simulink model "PTC_MBDS_StringDelete_Sample"  (R2013a)
settings: Solver=FixedStepDiscrete  StartTime=0.0  StopTime=100  FixedStep=0.02  RelTol=1e-3
libraries: PTC_MBDS_LIB x12, simulink_extras x1
settings Model: Creator=uidl7367  LastModifiedBy=sundeep.tuteja
settings DataIOCC: SignalLoggingSaveFormat=ModelDataLogs
settings OptimizationCC: ExpressionDepthLimit=2147483647  InitFltsAndDblsToZero=on
settings DebuggingCC: SaveWithParameterizedLinksMsg=none  SignalResolutionControl=TryResolveAllWithWarning  InheritedTsInSrcMsg=none  MultiTaskDSMMsg=warning  MultiTaskCondExecSysMsg=none  FcnCallInpInsideContextMsg=UseLocalSettings  StrictBusMsg=Warning
settings RTWCC: IncludeERTFirstTime=on
settings GRTTargetCC: TargetFcnLib=ansi_tfl_tmw.mat  CombineOutputUpdateFcns=off  GRTInterface=on

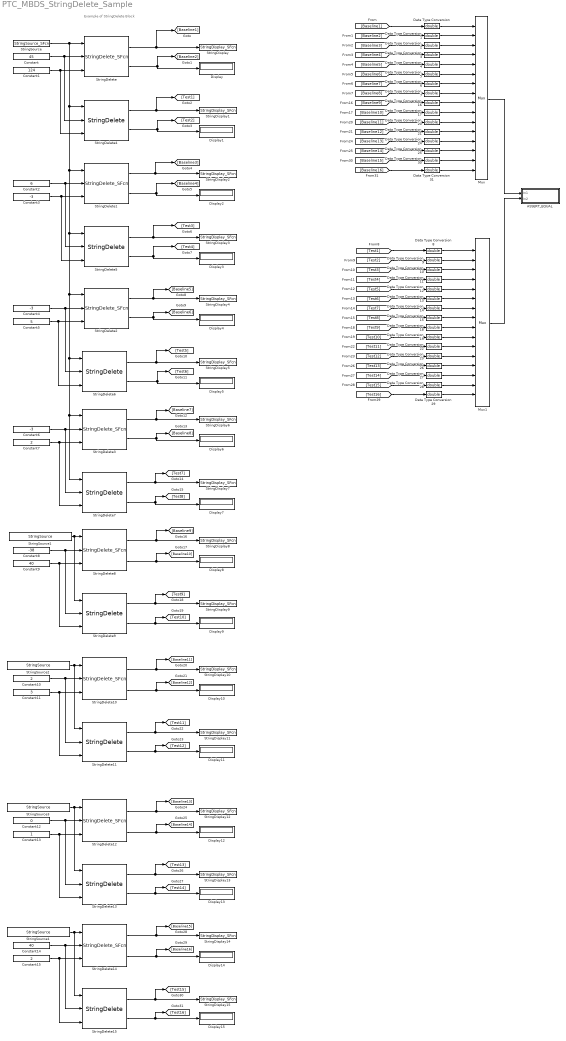
== system PTC_MBDS_StringDelete_Sample ==
  note: Example of StringDelete Block
  ASSERT_EQUAL : Subsystem
  Constant : Constant  InitFcn=|  Value=45  VectorParams1D=off  OutDataTypeStr=int8
      | if(exist('MBDS_BlockCallback', 'file'))
      |    MBDS_BlockCallback('Update', gcb);  
      | end
  Constant1 : Constant  InitFcn=|  Value=124  VectorParams1D=off  OutDataTypeStr=int8
      | if(exist('MBDS_BlockCallback', 'file'))
      |    MBDS_BlockCallback('Update', gcb);  
      | end
  Constant10 : Constant  InitFcn=|  Value=2  VectorParams1D=off  OutDataTypeStr=int8
      | if(exist('MBDS_BlockCallback', 'file'))
      |    MBDS_BlockCallback('Update', gcb);  
      | end
  Constant11 : Constant  InitFcn=|  Value=3  VectorParams1D=off  OutDataTypeStr=int8
      | if(exist('MBDS_BlockCallback', 'file'))
      |    MBDS_BlockCallback('Update', gcb);  
      | end
  Constant12 : Constant  InitFcn=|  Value=0  VectorParams1D=off  OutDataTypeStr=int8
      | if(exist('MBDS_BlockCallback', 'file'))
      |    MBDS_BlockCallback('Update', gcb);  
      | end
  Constant13 : Constant  InitFcn=|  VectorParams1D=off  OutDataTypeStr=int8
      | if(exist('MBDS_BlockCallback', 'file'))
      |    MBDS_BlockCallback('Update', gcb);  
      | end
  Constant14 : Constant  InitFcn=|  Value=40  VectorParams1D=off  OutDataTypeStr=int8
      | if(exist('MBDS_BlockCallback', 'file'))
      |    MBDS_BlockCallback('Update', gcb);  
      | end
  Constant15 : Constant  InitFcn=|  Value=2  VectorParams1D=off  OutDataTypeStr=int8
      | if(exist('MBDS_BlockCallback', 'file'))
      |    MBDS_BlockCallback('Update', gcb);  
      | end
  Constant2 : Constant  InitFcn=|  Value=6  VectorParams1D=off  OutDataTypeStr=int8
      | if(exist('MBDS_BlockCallback', 'file'))
      |    MBDS_BlockCallback('Update', gcb);  
      | end
  Constant3 : Constant  InitFcn=|  Value=-3  VectorParams1D=off  OutDataTypeStr=int8
      | if(exist('MBDS_BlockCallback', 'file'))
      |    MBDS_BlockCallback('Update', gcb);  
      | end
  Constant4 : Constant  InitFcn=|  Value=-3  VectorParams1D=off  OutDataTypeStr=int8
      | if(exist('MBDS_BlockCallback', 'file'))
      |    MBDS_BlockCallback('Update', gcb);  
      | end
  Constant5 : Constant  InitFcn=|  Value=5  VectorParams1D=off  OutDataTypeStr=int8
      | if(exist('MBDS_BlockCallback', 'file'))
      |    MBDS_BlockCallback('Update', gcb);  
      | end
  Constant6 : Constant  InitFcn=|  Value=-3  VectorParams1D=off  OutDataTypeStr=int8
      | if(exist('MBDS_BlockCallback', 'file'))
      |    MBDS_BlockCallback('Update', gcb);  
      | end
  Constant7 : Constant  InitFcn=|  Value=2  VectorParams1D=off  OutDataTypeStr=int8
      | if(exist('MBDS_BlockCallback', 'file'))
      |    MBDS_BlockCallback('Update', gcb);  
      | end
  Constant8 : Constant  InitFcn=|  Value=-38  VectorParams1D=off  OutDataTypeStr=int8
      | if(exist('MBDS_BlockCallback', 'file'))
      |    MBDS_BlockCallback('Update', gcb);  
      | end
  Constant9 : Constant  InitFcn=|  Value=40  VectorParams1D=off  OutDataTypeStr=int8
      | if(exist('MBDS_BlockCallback', 'file'))
      |    MBDS_BlockCallback('Update', gcb);  
      | end
  Data Type Conversion{,1..31} (32 alike) : DataTypeConversion  OutDataTypeStr=double
  Display{,1..15} (16 alike) : Display
  Mux : Mux  Inputs=16
  Mux1 : Mux  Inputs=16
  StringDelete : S-Function  InitFcn=|  FunctionName=StringDelete_SFcn  Parameters=boolean(ENO_Enabled), uint16(MaxStringLength)  EnableBusSupport=off  mask(StringDelete){MBDS_LibraryBlock=on, ENO_Enabled=on, MBDS_BlockVersion=05.40}
      | if(exist('MBDS_BlockCallback', 'file'))
      |    MBDS_BlockCallback('Update', gcb);
      | end
      mask prompts: MBDS_LibraryBlock "MBDS Library Block"; ENO_Enabled "Show ENO port"; MBDS_BlockVersion "Block version:"
      mask help: Removes a part of the string at input port In. The first character to be removed is given by P, the number of characters to be removed is given by L.
      mask init:
      | MBDS_BlockCallback('Copy', gcb);
      | MaxStringLength = 1 + GetStringLen();
      | maskdisplay = ['disp(''Delete'')' 10];
      | maskdisplay = [maskdisplay 'port_label(''input'', 1, ''In'')' 10];
      | maskdisplay = [maskdisplay 'port_label(''input'', 2, ''L'')' 10];
      | maskdisplay = [maskdisplay 'port_label(''input'', 3, ''P'')' 10];
      | maskdisplay = [maskdisplay 'port_label(''output'', 1, ''Out'')' 10];
      | if(ENO_Enabled)
      | 	maskdisplay = [maskdisplay 'port_label(''output'', 2, ''ENO'')' 10];
      | end
      | set_param(gcbh, 'maskdisplay', maskdisplay)
      mask Help: eval(['open([workdir(''Library_Dir:''),''\Blockset\Help\'',get_param(gcb,''MaskType''),''.html''])'])
      mask Display:
      | disp('Delete')
      | port_label('input', 1, 'In')
      | port_label('input', 2, 'L')
      | port_label('input', 3, 'P')
      | port_label('output', 1, 'Out')
      | port_label('output', 2, 'ENO')
  StringDelete1 : S-Function  InitFcn=|  FunctionName=StringDelete_SFcn  Parameters=boolean(ENO_Enabled), uint16(MaxStringLength)  EnableBusSupport=off  mask(StringDelete){MBDS_LibraryBlock=on, ENO_Enabled=on, MBDS_BlockVersion=05.40}
      | if(exist('MBDS_BlockCallback', 'file'))
      |    MBDS_BlockCallback('Update', gcb);
      | end
      mask prompts: MBDS_LibraryBlock "MBDS Library Block"; ENO_Enabled "Show ENO port"; MBDS_BlockVersion "Block version:"
      mask help: Removes a part of the string at input port In. The first character to be removed is given by P, the number of characters to be removed is given by L.
      mask init: same as PTC_MBDS_StringDelete_Sample/StringDelete
      mask Help: eval(['open([workdir(''Library_Dir:''),''\Blockset\Help\'',get_param(gcb,''MaskType''),''.html''])'])
      mask Display:
      | disp('Delete')
      | port_label('input', 1, 'In')
      | port_label('input', 2, 'L')
      | port_label('input', 3, 'P')
      | port_label('output', 1, 'Out')
      | port_label('output', 2, 'ENO')
  StringDelete10 : S-Function  InitFcn=|  FunctionName=StringDelete_SFcn  Parameters=boolean(ENO_Enabled), uint16(MaxStringLength)  EnableBusSupport=off  mask(StringDelete){MBDS_LibraryBlock=on, ENO_Enabled=on, MBDS_BlockVersion=05.32}
      | if(exist('MBDS_BlockCallback', 'file'))
      |    MBDS_BlockCallback('Update', gcb);
      | end
      mask prompts: MBDS_LibraryBlock "MBDS Library Block"; ENO_Enabled "Show ENO port"; MBDS_BlockVersion "Block version:"
      mask help: Removes a part of the string at input port In. The first character to be removed is given by P, the number of characters to be removed is given by L.
      mask init: same as PTC_MBDS_StringDelete_Sample/StringDelete
      mask Help: eval(['open([workdir(''Library_Dir:''),''\Blockset\Help\'',get_param(gcb,''MaskType''),''.html''])'])
      mask Display:
      | disp('Delete')
      | port_label('input', 1, 'In')
      | port_label('input', 2, 'L')
      | port_label('input', 3, 'P')
      | port_label('output', 1, 'Out')
      | port_label('output', 2, 'ENO')
  StringDelete{4..7,9,11,13,15} (8 alike) : PTC_MBDS_LIB/MBDS Standard Library/Extended Operations/String Operations/StringDelete  ENO_Enabled=on  MaxStringLength=PTC_MBDS_MaxStringLength_Fcn  PTC_MBDS_BlockVersion=5.32  PTC_BlockType=PTC_MBDS_StringDelete
  StringDelete12 : S-Function  InitFcn=|  FunctionName=StringDelete_SFcn  Parameters=boolean(ENO_Enabled), uint16(MaxStringLength)  EnableBusSupport=off  mask(StringDelete){MBDS_LibraryBlock=on, ENO_Enabled=on, MBDS_BlockVersion=05.32}
      | if(exist('MBDS_BlockCallback', 'file'))
      |    MBDS_BlockCallback('Update', gcb);
      | end
      mask prompts: MBDS_LibraryBlock "MBDS Library Block"; ENO_Enabled "Show ENO port"; MBDS_BlockVersion "Block version:"
      mask help: Removes a part of the string at input port In. The first character to be removed is given by P, the number of characters to be removed is given by L.
      mask init: same as PTC_MBDS_StringDelete_Sample/StringDelete
      mask Help: eval(['open([workdir(''Library_Dir:''),''\Blockset\Help\'',get_param(gcb,''MaskType''),''.html''])'])
      mask Display:
      | disp('Delete')
      | port_label('input', 1, 'In')
      | port_label('input', 2, 'L')
      | port_label('input', 3, 'P')
      | port_label('output', 1, 'Out')
      | port_label('output', 2, 'ENO')
  StringDelete14 : S-Function  InitFcn=|  FunctionName=StringDelete_SFcn  Parameters=boolean(ENO_Enabled), uint16(MaxStringLength)  EnableBusSupport=off  mask(StringDelete){MBDS_LibraryBlock=on, ENO_Enabled=on, MBDS_BlockVersion=05.32}
      | if(exist('MBDS_BlockCallback', 'file'))
      |    MBDS_BlockCallback('Update', gcb);
      | end
      mask prompts: MBDS_LibraryBlock "MBDS Library Block"; ENO_Enabled "Show ENO port"; MBDS_BlockVersion "Block version:"
      mask help: Removes a part of the string at input port In. The first character to be removed is given by P, the number of characters to be removed is given by L.
      mask init: same as PTC_MBDS_StringDelete_Sample/StringDelete
      mask Help: eval(['open([workdir(''Library_Dir:''),''\Blockset\Help\'',get_param(gcb,''MaskType''),''.html''])'])
      mask Display:
      | disp('Delete')
      | port_label('input', 1, 'In')
      | port_label('input', 2, 'L')
      | port_label('input', 3, 'P')
      | port_label('output', 1, 'Out')
      | port_label('output', 2, 'ENO')
  StringDelete2 : S-Function  InitFcn=|  FunctionName=StringDelete_SFcn  Parameters=boolean(ENO_Enabled), uint16(MaxStringLength)  EnableBusSupport=off  mask(StringDelete){MBDS_LibraryBlock=on, ENO_Enabled=on, MBDS_BlockVersion=05.40}
      | if(exist('MBDS_BlockCallback', 'file'))
      |    MBDS_BlockCallback('Update', gcb);
      | end
      mask prompts: MBDS_LibraryBlock "MBDS Library Block"; ENO_Enabled "Show ENO port"; MBDS_BlockVersion "Block version:"
      mask help: Removes a part of the string at input port In. The first character to be removed is given by P, the number of characters to be removed is given by L.
      mask init: same as PTC_MBDS_StringDelete_Sample/StringDelete
      mask Help: eval(['open([workdir(''Library_Dir:''),''\Blockset\Help\'',get_param(gcb,''MaskType''),''.html''])'])
      mask Display:
      | disp('Delete')
      | port_label('input', 1, 'In')
      | port_label('input', 2, 'L')
      | port_label('input', 3, 'P')
      | port_label('output', 1, 'Out')
      | port_label('output', 2, 'ENO')
  StringDelete3 : S-Function  InitFcn=|  FunctionName=StringDelete_SFcn  Parameters=boolean(ENO_Enabled), uint16(MaxStringLength)  EnableBusSupport=off  mask(StringDelete){MBDS_LibraryBlock=on, ENO_Enabled=on, MBDS_BlockVersion=05.40}
      | if(exist('MBDS_BlockCallback', 'file'))
      |    MBDS_BlockCallback('Update', gcb);
      | end
      mask prompts: MBDS_LibraryBlock "MBDS Library Block"; ENO_Enabled "Show ENO port"; MBDS_BlockVersion "Block version:"
      mask help: Removes a part of the string at input port In. The first character to be removed is given by P, the number of characters to be removed is given by L.
      mask init: same as PTC_MBDS_StringDelete_Sample/StringDelete
      mask Help: eval(['open([workdir(''Library_Dir:''),''\Blockset\Help\'',get_param(gcb,''MaskType''),''.html''])'])
      mask Display:
      | disp('Delete')
      | port_label('input', 1, 'In')
      | port_label('input', 2, 'L')
      | port_label('input', 3, 'P')
      | port_label('output', 1, 'Out')
      | port_label('output', 2, 'ENO')
  StringDelete8 : S-Function  InitFcn=|  FunctionName=StringDelete_SFcn  Parameters=boolean(ENO_Enabled), uint16(MaxStringLength)  EnableBusSupport=off  mask(StringDelete){MBDS_LibraryBlock=on, ENO_Enabled=on, MBDS_BlockVersion=05.32}
      | if(exist('MBDS_BlockCallback', 'file'))
      |    MBDS_BlockCallback('Update', gcb);
      | end
      mask prompts: MBDS_LibraryBlock "MBDS Library Block"; ENO_Enabled "Show ENO port"; MBDS_BlockVersion "Block version:"
      mask help: Removes a part of the string at input port In. The first character to be removed is given by P, the number of characters to be removed is given by L.
      mask init: same as PTC_MBDS_StringDelete_Sample/StringDelete
      mask Help: eval(['open([workdir(''Library_Dir:''),''\Blockset\Help\'',get_param(gcb,''MaskType''),''.html''])'])
      mask Display:
      | disp('Delete')
      | port_label('input', 1, 'In')
      | port_label('input', 2, 'L')
      | port_label('input', 3, 'P')
      | port_label('output', 1, 'Out')
      | port_label('output', 2, 'ENO')
  StringDisplay : M-S-Function  InitFcn=|  FunctionName=StringDisplay_SFcn  Parameters=MaxRowCount  mask(StringDisplay){MBDS_LibraryBlock=on, MaxRowCount=1, MBDS_BlockVersion=05.20}
      | if(exist('MBDS_BlockCallback', 'file'))
      |    MBDS_BlockCallback('Update', gcb);
      | end
      mask prompts: MBDS_LibraryBlock "MBDS Library Block"; MaxRowCount "Maximum number of rows displayed (min. 1):"; MBDS_BlockVersion "Block version:"
      mask help: The string display block shows an uint8 array as ASCII strings on the block mask.
      mask init:
      | MBDS_BlockCallback('Copy', gcb);
      mask Help: eval(['open([workdir(''Library_Dir:''),''\Blockset\Help\'',get_param(gcb,''MaskType''),''.html''])'])
      mask Callback MaxRowCount:
      | if(str2double(get_param(gcb, 'MaxRowCount')) < 1)
      |    set_param(gcb, 'MaxRowCount', '1');
      | end
      mask Display: text(0.05,0.5,'40_character_string_00000000000000000000','horizontalAlignment','left','verticalAlignment','middle')
  StringDisplay1 : M-S-Function  InitFcn=|  FunctionName=StringDisplay_SFcn  Parameters=MaxRowCount  mask(StringDisplay){MBDS_LibraryBlock=on, MaxRowCount=1, MBDS_BlockVersion=05.20}
      | if(exist('MBDS_BlockCallback', 'file'))
      |    MBDS_BlockCallback('Update', gcb);
      | end
      mask prompts: MBDS_LibraryBlock "MBDS Library Block"; MaxRowCount "Maximum number of rows displayed (min. 1):"; MBDS_BlockVersion "Block version:"
      mask help: The string display block shows an uint8 array as ASCII strings on the block mask.
      mask init:
      | MBDS_BlockCallback('Copy', gcb);
      mask Help: eval(['open([workdir(''Library_Dir:''),''\Blockset\Help\'',get_param(gcb,''MaskType''),''.html''])'])
      mask Callback MaxRowCount:
      | if(str2double(get_param(gcb, 'MaxRowCount')) < 1)
      |    set_param(gcb, 'MaxRowCount', '1');
      | end
      mask Display: text(0.05,0.5,'40_character_string_00000000000000000000','horizontalAlignment','left','verticalAlignment','middle')
  StringDisplay10 : M-S-Function  InitFcn=|  FunctionName=StringDisplay_SFcn  Parameters=MaxRowCount  mask(StringDisplay){MBDS_LibraryBlock=on, MaxRowCount=1, MBDS_BlockVersion=05.20}
      | if(exist('MBDS_BlockCallback', 'file'))
      |    MBDS_BlockCallback('Update', gcb);
      | end
      mask prompts: MBDS_LibraryBlock "MBDS Library Block"; MaxRowCount "Maximum number of rows displayed (min. 1):"; MBDS_BlockVersion "Block version:"
      mask help: The string display block shows an uint8 array as ASCII strings on the block mask.
      mask init:
      | MBDS_BlockCallback('Copy', gcb);
      mask Help: eval(['open([workdir(''Library_Dir:''),''\Blockset\Help\'',get_param(gcb,''MaskType''),''.html''])'])
      mask Callback MaxRowCount:
      | if(str2double(get_param(gcb, 'MaxRowCount')) < 1)
      |    set_param(gcb, 'MaxRowCount', '1');
      | end
      mask Display: text(0.05,0.5,'Myring','horizontalAlignment','left','verticalAlignment','middle')
  StringDisplay11 : M-S-Function  InitFcn=|  FunctionName=StringDisplay_SFcn  Parameters=MaxRowCount  mask(StringDisplay){MBDS_LibraryBlock=on, MaxRowCount=1, MBDS_BlockVersion=05.20}
      | if(exist('MBDS_BlockCallback', 'file'))
      |    MBDS_BlockCallback('Update', gcb);
      | end
      mask prompts: MBDS_LibraryBlock "MBDS Library Block"; MaxRowCount "Maximum number of rows displayed (min. 1):"; MBDS_BlockVersion "Block version:"
      mask help: The string display block shows an uint8 array as ASCII strings on the block mask.
      mask init:
      | MBDS_BlockCallback('Copy', gcb);
      mask Help: eval(['open([workdir(''Library_Dir:''),''\Blockset\Help\'',get_param(gcb,''MaskType''),''.html''])'])
      mask Callback MaxRowCount:
      | if(str2double(get_param(gcb, 'MaxRowCount')) < 1)
      |    set_param(gcb, 'MaxRowCount', '1');
      | end
      mask Display: text(0.05,0.5,'Myring','horizontalAlignment','left','verticalAlignment','middle')
  StringDisplay12 : M-S-Function  InitFcn=|  FunctionName=StringDisplay_SFcn  Parameters=MaxRowCount  mask(StringDisplay){MBDS_LibraryBlock=on, MaxRowCount=1, MBDS_BlockVersion=05.20}
      | if(exist('MBDS_BlockCallback', 'file'))
      |    MBDS_BlockCallback('Update', gcb);
      | end
      mask prompts: MBDS_LibraryBlock "MBDS Library Block"; MaxRowCount "Maximum number of rows displayed (min. 1):"; MBDS_BlockVersion "Block version:"
      mask help: The string display block shows an uint8 array as ASCII strings on the block mask.
      mask init:
      | MBDS_BlockCallback('Copy', gcb);
      mask Help: eval(['open([workdir(''Library_Dir:''),''\Blockset\Help\'',get_param(gcb,''MaskType''),''.html''])'])
      mask Callback MaxRowCount:
      | if(str2double(get_param(gcb, 'MaxRowCount')) < 1)
      |    set_param(gcb, 'MaxRowCount', '1');
      | end
      mask Display: text(0.05,0.5,'38NrfmUQH0DuKObcdee8fC8Gn_9QencF7KBLnQuN','horizontalAlignment','left','verticalAlignment','middle')
  StringDisplay13 : M-S-Function  InitFcn=|  FunctionName=StringDisplay_SFcn  Parameters=MaxRowCount  mask(StringDisplay){MBDS_LibraryBlock=on, MaxRowCount=1, MBDS_BlockVersion=05.20}
      | if(exist('MBDS_BlockCallback', 'file'))
      |    MBDS_BlockCallback('Update', gcb);
      | end
      mask prompts: MBDS_LibraryBlock "MBDS Library Block"; MaxRowCount "Maximum number of rows displayed (min. 1):"; MBDS_BlockVersion "Block version:"
      mask help: The string display block shows an uint8 array as ASCII strings on the block mask.
      mask init:
      | MBDS_BlockCallback('Copy', gcb);
      mask Help: eval(['open([workdir(''Library_Dir:''),''\Blockset\Help\'',get_param(gcb,''MaskType''),''.html''])'])
      mask Callback MaxRowCount:
      | if(str2double(get_param(gcb, 'MaxRowCount')) < 1)
      |    set_param(gcb, 'MaxRowCount', '1');
      | end
      mask Display: text(0.05,0.5,'38NrfmUQH0DuKObcdee8fC8Gn_9QencF7KBLnQuN','horizontalAlignment','left','verticalAlignment','middle')
  StringDisplay14 : M-S-Function  InitFcn=|  FunctionName=StringDisplay_SFcn  Parameters=MaxRowCount  mask(StringDisplay){MBDS_LibraryBlock=on, MaxRowCount=1, MBDS_BlockVersion=05.20}
      | if(exist('MBDS_BlockCallback', 'file'))
      |    MBDS_BlockCallback('Update', gcb);
      | end
      mask prompts: MBDS_LibraryBlock "MBDS Library Block"; MaxRowCount "Maximum number of rows displayed (min. 1):"; MBDS_BlockVersion "Block version:"
      mask help: The string display block shows an uint8 array as ASCII strings on the block mask.
      mask init:
      | MBDS_BlockCallback('Copy', gcb);
      mask Help: eval(['open([workdir(''Library_Dir:''),''\Blockset\Help\'',get_param(gcb,''MaskType''),''.html''])'])
      mask Callback MaxRowCount:
      | if(str2double(get_param(gcb, 'MaxRowCount')) < 1)
      |    set_param(gcb, 'MaxRowCount', '1');
      | end
      mask Display: text(0.05,0.5,'38NrfmUQH0DuKObcdee8fC8Gn_9QencF7KBLnQuN','horizontalAlignment','left','verticalAlignment','middle')
  StringDisplay15 : M-S-Function  InitFcn=|  FunctionName=StringDisplay_SFcn  Parameters=MaxRowCount  mask(StringDisplay){MBDS_LibraryBlock=on, MaxRowCount=1, MBDS_BlockVersion=05.20}
      | if(exist('MBDS_BlockCallback', 'file'))
      |    MBDS_BlockCallback('Update', gcb);
      | end
      mask prompts: MBDS_LibraryBlock "MBDS Library Block"; MaxRowCount "Maximum number of rows displayed (min. 1):"; MBDS_BlockVersion "Block version:"
      mask help: The string display block shows an uint8 array as ASCII strings on the block mask.
      mask init:
      | MBDS_BlockCallback('Copy', gcb);
      mask Help: eval(['open([workdir(''Library_Dir:''),''\Blockset\Help\'',get_param(gcb,''MaskType''),''.html''])'])
      mask Callback MaxRowCount:
      | if(str2double(get_param(gcb, 'MaxRowCount')) < 1)
      |    set_param(gcb, 'MaxRowCount', '1');
      | end
      mask Display: text(0.05,0.5,'38NrfmUQH0DuKObcdee8fC8Gn_9QencF7KBLnQuN','horizontalAlignment','left','verticalAlignment','middle')
  StringDisplay2 : M-S-Function  InitFcn=|  FunctionName=StringDisplay_SFcn  Parameters=MaxRowCount  mask(StringDisplay){MBDS_LibraryBlock=on, MaxRowCount=1, MBDS_BlockVersion=05.20}
      | if(exist('MBDS_BlockCallback', 'file'))
      |    MBDS_BlockCallback('Update', gcb);
      | end
      mask prompts: MBDS_LibraryBlock "MBDS Library Block"; MaxRowCount "Maximum number of rows displayed (min. 1):"; MBDS_BlockVersion "Block version:"
      mask help: The string display block shows an uint8 array as ASCII strings on the block mask.
      mask init:
      | MBDS_BlockCallback('Copy', gcb);
      mask Help: eval(['open([workdir(''Library_Dir:''),''\Blockset\Help\'',get_param(gcb,''MaskType''),''.html''])'])
      mask Callback MaxRowCount:
      | if(str2double(get_param(gcb, 'MaxRowCount')) < 1)
      |    set_param(gcb, 'MaxRowCount', '1');
      | end
      mask Display: text(0.05,0.5,'_character_string_00000000000000000000','horizontalAlignment','left','verticalAlignment','middle')
  StringDisplay3 : M-S-Function  InitFcn=|  FunctionName=StringDisplay_SFcn  Parameters=MaxRowCount  mask(StringDisplay){MBDS_LibraryBlock=on, MaxRowCount=1, MBDS_BlockVersion=05.20}
      | if(exist('MBDS_BlockCallback', 'file'))
      |    MBDS_BlockCallback('Update', gcb);
      | end
      mask prompts: MBDS_LibraryBlock "MBDS Library Block"; MaxRowCount "Maximum number of rows displayed (min. 1):"; MBDS_BlockVersion "Block version:"
      mask help: The string display block shows an uint8 array as ASCII strings on the block mask.
      mask init:
      | MBDS_BlockCallback('Copy', gcb);
      mask Help: eval(['open([workdir(''Library_Dir:''),''\Blockset\Help\'',get_param(gcb,''MaskType''),''.html''])'])
      mask Callback MaxRowCount:
      | if(str2double(get_param(gcb, 'MaxRowCount')) < 1)
      |    set_param(gcb, 'MaxRowCount', '1');
      | end
      mask Display: text(0.05,0.5,'_character_string_00000000000000000000','horizontalAlignment','left','verticalAlignment','middle')
  StringDisplay4 : M-S-Function  InitFcn=|  FunctionName=StringDisplay_SFcn  Parameters=MaxRowCount  mask(StringDisplay){MBDS_LibraryBlock=on, MaxRowCount=1, MBDS_BlockVersion=05.20}
      | if(exist('MBDS_BlockCallback', 'file'))
      |    MBDS_BlockCallback('Update', gcb);
      | end
      mask prompts: MBDS_LibraryBlock "MBDS Library Block"; MaxRowCount "Maximum number of rows displayed (min. 1):"; MBDS_BlockVersion "Block version:"
      mask help: The string display block shows an uint8 array as ASCII strings on the block mask.
      mask init:
      | MBDS_BlockCallback('Copy', gcb);
      mask Help: eval(['open([workdir(''Library_Dir:''),''\Blockset\Help\'',get_param(gcb,''MaskType''),''.html''])'])
      mask Callback MaxRowCount:
      | if(str2double(get_param(gcb, 'MaxRowCount')) < 1)
      |    set_param(gcb, 'MaxRowCount', '1');
      | end
      mask Display: text(0.05,0.5,'4haracter_string_00000000000000000000','horizontalAlignment','left','verticalAlignment','middle')
  StringDisplay5 : M-S-Function  InitFcn=|  FunctionName=StringDisplay_SFcn  Parameters=MaxRowCount  mask(StringDisplay){MBDS_LibraryBlock=on, MaxRowCount=1, MBDS_BlockVersion=05.20}
      | if(exist('MBDS_BlockCallback', 'file'))
      |    MBDS_BlockCallback('Update', gcb);
      | end
      mask prompts: MBDS_LibraryBlock "MBDS Library Block"; MaxRowCount "Maximum number of rows displayed (min. 1):"; MBDS_BlockVersion "Block version:"
      mask help: The string display block shows an uint8 array as ASCII strings on the block mask.
      mask init:
      | MBDS_BlockCallback('Copy', gcb);
      mask Help: eval(['open([workdir(''Library_Dir:''),''\Blockset\Help\'',get_param(gcb,''MaskType''),''.html''])'])
      mask Callback MaxRowCount:
      | if(str2double(get_param(gcb, 'MaxRowCount')) < 1)
      |    set_param(gcb, 'MaxRowCount', '1');
      | end
      mask Display: text(0.05,0.5,'4haracter_string_00000000000000000000','horizontalAlignment','left','verticalAlignment','middle')
  StringDisplay6 : M-S-Function  InitFcn=|  FunctionName=StringDisplay_SFcn  Parameters=MaxRowCount  mask(StringDisplay){MBDS_LibraryBlock=on, MaxRowCount=1, MBDS_BlockVersion=05.20}
      | if(exist('MBDS_BlockCallback', 'file'))
      |    MBDS_BlockCallback('Update', gcb);
      | end
      mask prompts: MBDS_LibraryBlock "MBDS Library Block"; MaxRowCount "Maximum number of rows displayed (min. 1):"; MBDS_BlockVersion "Block version:"
      mask help: The string display block shows an uint8 array as ASCII strings on the block mask.
      mask init:
      | MBDS_BlockCallback('Copy', gcb);
      mask Help: eval(['open([workdir(''Library_Dir:''),''\Blockset\Help\'',get_param(gcb,''MaskType''),''.html''])'])
      mask Callback MaxRowCount:
      | if(str2double(get_param(gcb, 'MaxRowCount')) < 1)
      |    set_param(gcb, 'MaxRowCount', '1');
      | end
      mask Display: text(0.05,0.5,'0_character_string_00000000000000000000','horizontalAlignment','left','verticalAlignment','middle')
  StringDisplay7 : M-S-Function  InitFcn=|  FunctionName=StringDisplay_SFcn  Parameters=MaxRowCount  mask(StringDisplay){MBDS_LibraryBlock=on, MaxRowCount=1, MBDS_BlockVersion=05.20}
      | if(exist('MBDS_BlockCallback', 'file'))
      |    MBDS_BlockCallback('Update', gcb);
      | end
      mask prompts: MBDS_LibraryBlock "MBDS Library Block"; MaxRowCount "Maximum number of rows displayed (min. 1):"; MBDS_BlockVersion "Block version:"
      mask help: The string display block shows an uint8 array as ASCII strings on the block mask.
      mask init:
      | MBDS_BlockCallback('Copy', gcb);
      mask Help: eval(['open([workdir(''Library_Dir:''),''\Blockset\Help\'',get_param(gcb,''MaskType''),''.html''])'])
      mask Callback MaxRowCount:
      | if(str2double(get_param(gcb, 'MaxRowCount')) < 1)
      |    set_param(gcb, 'MaxRowCount', '1');
      | end
      mask Display: text(0.05,0.5,'0_character_string_00000000000000000000','horizontalAlignment','left','verticalAlignment','middle')
  StringDisplay8 : M-S-Function  InitFcn=|  FunctionName=StringDisplay_SFcn  Parameters=MaxRowCount  mask(StringDisplay){MBDS_LibraryBlock=on, MaxRowCount=1, MBDS_BlockVersion=05.20}
      | if(exist('MBDS_BlockCallback', 'file'))
      |    MBDS_BlockCallback('Update', gcb);
      | end
      mask prompts: MBDS_LibraryBlock "MBDS Library Block"; MaxRowCount "Maximum number of rows displayed (min. 1):"; MBDS_BlockVersion "Block version:"
      mask help: The string display block shows an uint8 array as ASCII strings on the block mask.
      mask init:
      | MBDS_BlockCallback('Copy', gcb);
      mask Help: eval(['open([workdir(''Library_Dir:''),''\Blockset\Help\'',get_param(gcb,''MaskType''),''.html''])'])
      mask Callback MaxRowCount:
      | if(str2double(get_param(gcb, 'MaxRowCount')) < 1)
      |    set_param(gcb, 'MaxRowCount', '1');
      | end
      mask Display: text(0.05,0.5,'a','horizontalAlignment','left','verticalAlignment','middle')
  StringDisplay9 : M-S-Function  InitFcn=|  FunctionName=StringDisplay_SFcn  Parameters=MaxRowCount  mask(StringDisplay){MBDS_LibraryBlock=on, MaxRowCount=1, MBDS_BlockVersion=05.20}
      | if(exist('MBDS_BlockCallback', 'file'))
      |    MBDS_BlockCallback('Update', gcb);
      | end
      mask prompts: MBDS_LibraryBlock "MBDS Library Block"; MaxRowCount "Maximum number of rows displayed (min. 1):"; MBDS_BlockVersion "Block version:"
      mask help: The string display block shows an uint8 array as ASCII strings on the block mask.
      mask init:
      | MBDS_BlockCallback('Copy', gcb);
      mask Help: eval(['open([workdir(''Library_Dir:''),''\Blockset\Help\'',get_param(gcb,''MaskType''),''.html''])'])
      mask Callback MaxRowCount:
      | if(str2double(get_param(gcb, 'MaxRowCount')) < 1)
      |    set_param(gcb, 'MaxRowCount', '1');
      | end
      mask Display: text(0.05,0.5,'a','horizontalAlignment','left','verticalAlignment','middle')
  StringSource : S-Function  InitFcn=|  FunctionName=StringSource_SFcn  Parameters=uint8(String), uint16(MaxStringLength)  EnableBusSupport=off  mask(StringSource){MBDS_LibraryBlock=on, InputValue=40_character_string_00000000000000000000, MBDS_BlockVersion=05.20}
      | if(exist('MBDS_BlockCallback', 'file'))
      |    MBDS_BlockCallback('Update', gcb);
      | end
      mask prompts: MBDS_LibraryBlock "MBDS Library Block"; InputValue "Constant value:"; MBDS_BlockVersion "Block version:"
      mask help: This block outputs an uint8 array based on the ASCII codes of the string specified by the user.
      mask init:
      | MBDS_BlockCallback('Copy', gcb);
      | MaxStringLength = 1 + GetStringLen();
      | DispString = 'Error';
      | String = InputValue;
      | % Skip if string specifies a numeric expression or starts with '
      | if(isempty(str2num(String)) && String(1) ~= '''')
      |    try
      |       % Try to evaluate project constant 
      |       String = evalin('base', String);
      |    end   
      | end
      | if ~ischar(String) || size(String, 1) > 1
      | 	error('String must be a [1xn] array of type ''char'' with at least one character')
      | else
      |    % Limit to max. string length
      |    String = String(1:min(MaxStringLength, length(String)));
      | 	DispString = InputValue;
      | end
      mask Help: eval(['open([workdir(''Library_Dir:''),''\Blockset\Help\'',get_param(gcb,''MaskType''),''.html''])'])
      mask Display: text(0.05,0.5,DispString,'horizontalAlignment','left')
  StringSource1 : PTC_MBDS_LIB/MBDS Standard Library/Extended Operations/String Operations/StringSource  InputValue=ab  PTC_MBDS_BlockVersion=5.32  PTC_BlockType=PTC_MBDS_StringSource  Value=uint8([97; 98; 0; 0; 0; 0; 0; 0; 0; 0; 0; 0; 0; 0; 0; 0; 0; 0; 0; 0; 0; 0; 0; 0; 0; 0; 0; 0; 0; 0; 0; 0; 0; 0; 0; 0; 0; 0; 0; 0; 0])  MaxStringLength=PTC_MBDS_MaxStringLength_Fcn
  StringSource2 : PTC_MBDS_LIB/MBDS Standard Library/Extended Operations/String Operations/StringSource  InputValue=MyString  PTC_MBDS_BlockVersion=5.32  PTC_BlockType=PTC_MBDS_StringSource  Value=uint8([77; 121; 83; 116; 114; 105; 110; 103; 0; 0; 0; 0; 0; 0; 0; 0; 0; 0; 0; 0; 0; 0; 0; 0; 0; 0; 0; 0; 0; 0; 0; 0; 0; 0; 0; 0; 0; 0; 0; 0; 0])  MaxStringLength=PTC_MBDS_MaxStringLength_Fcn
  StringSource3 : PTC_MBDS_LIB/MBDS Standard Library/Extended Operations/String Operations/StringSource  InputValue=38NrfmUQH0DuKObcdee8fC8Gn_9QencF7KBLnQuN  PTC_MBDS_BlockVersion=5.32  PTC_BlockType=PTC_MBDS_StringSource  Value=uint8([51; 56; 78; 114; 102; 109; 85; 81; 72; 48; 68; 117; 75; 79; 98; 99; 100; 101; 101; 56; 102; 67; 56; 71; 110; 95; 57; 81; 101; 110; 99; 70; 55; 75; 66; 76; 110; 81; 117; 78; 0])  MaxStringLength=PTC_MBDS_MaxStringLength_Fcn
  StringSource4 : PTC_MBDS_LIB/MBDS Standard Library/Extended Operations/String Operations/StringSource  InputValue=BLtTv9AEOWql9YuunQmrOgfUvMDVNs6EgZ5NvIfv  PTC_MBDS_BlockVersion=5.32  PTC_BlockType=PTC_MBDS_StringSource  Value=uint8([66; 76; 116; 84; 118; 57; 65; 69; 79; 87; 113; 108; 57; 89; 117; 117; 110; 81; 109; 114; 79; 103; 102; 85; 118; 77; 68; 86; 78; 115; 54; 69; 103; 90; 53; 78; 118; 73; 102; 118; 0])  MaxStringLength=PTC_MBDS_MaxStringLength_Fcn
  wires:
  StringSource/1 -> StringDelete4/1, StringDelete7/1, StringDelete3/1, StringDelete6/1, StringDelete2/1, StringDelete5/1, StringDelete1/1, StringDelete/1
  StringDelete/1 -> [Baseline1], StringDisplay/1
  Constant/1 -> StringDelete4/2, StringDelete/2
  Constant1/1 -> StringDelete4/3, StringDelete/3
  StringDelete/2 -> Display/1, [Baseline2]
  StringDelete4/1 -> [Test1], StringDisplay1/1
  StringDelete4/2 -> Display1/1, [Test2]
  StringDelete1/1 -> [Baseline3], StringDisplay2/1
  StringDelete1/2 -> Display2/1, [Baseline4]
  StringDelete5/1 -> [Test3], StringDisplay3/1
  StringDelete5/2 -> Display3/1, [Test4]
  Constant2/1 -> StringDelete5/2, StringDelete1/2
  Constant3/1 -> StringDelete5/3, StringDelete1/3
  StringDelete2/1 -> [Baseline5], StringDisplay4/1
  StringDelete2/2 -> Display4/1, [Baseline6]
  StringDelete6/1 -> [Test5], StringDisplay5/1
  StringDelete6/2 -> Display5/1, [Test6]
  Constant4/1 -> StringDelete6/2, StringDelete2/2
  Constant5/1 -> StringDelete6/3, StringDelete2/3
  StringDelete3/1 -> [Baseline7], StringDisplay6/1
  StringDelete3/2 -> Display6/1, [Baseline8]
  StringDelete7/1 -> [Test7], StringDisplay7/1
  StringDelete7/2 -> Display7/1, [Test8]
  Constant6/1 -> StringDelete7/2, StringDelete3/2
  Constant7/1 -> StringDelete7/3, StringDelete3/3
  Mux/1 -> ASSERT_EQUAL/1(In1)
  Mux1/1 -> ASSERT_EQUAL/2(In2)
  [Baseline6] -> Data Type Conversion5/1
  [Baseline2] -> Data Type Conversion1/1
  [Baseline4] -> Data Type Conversion3/1
  [Baseline5] -> Data Type Conversion4/1
  [Baseline3] -> Data Type Conversion2/1
  [Baseline8] -> Data Type Conversion7/1
  [Baseline7] -> Data Type Conversion6/1
  [Baseline1] -> Data Type Conversion/1
  [Test6] -> Data Type Conversion13/1
  [Test8] -> Data Type Conversion15/1
  [Test1] -> Data Type Conversion8/1
  [Test4] -> Data Type Conversion11/1
  [Test5] -> Data Type Conversion12/1
  [Test7] -> Data Type Conversion14/1
  [Test3] -> Data Type Conversion10/1
  [Test2] -> Data Type Conversion9/1
  Data Type Conversion/1 -> Mux/1
  Data Type Conversion1/1 -> Mux/2
  Data Type Conversion2/1 -> Mux/3
  Data Type Conversion3/1 -> Mux/4
  Data Type Conversion4/1 -> Mux/5
  Data Type Conversion5/1 -> Mux/6
  Data Type Conversion6/1 -> Mux/7
  Data Type Conversion7/1 -> Mux/8
  Data Type Conversion8/1 -> Mux1/1
  Data Type Conversion9/1 -> Mux1/2
  Data Type Conversion10/1 -> Mux1/3
  Data Type Conversion11/1 -> Mux1/4
  Data Type Conversion12/1 -> Mux1/5
  Data Type Conversion13/1 -> Mux1/6
  Data Type Conversion14/1 -> Mux1/7
  Data Type Conversion15/1 -> Mux1/8
  StringDelete8/1 -> [Baseline9], StringDisplay8/1
  StringDelete8/2 -> [Baseline10], Display8/1
  StringDelete9/1 -> [Test9], StringDisplay9/1
  StringDelete9/2 -> Display9/1, [Test10]
  Constant8/1 -> StringDelete9/2, StringDelete8/2
  Constant9/1 -> StringDelete9/3, StringDelete8/3
  StringSource1/1 -> StringDelete9/1, StringDelete8/1
  [Baseline9] -> Data Type Conversion16/1
  Data Type Conversion16/1 -> Mux/9
  [Baseline10] -> Data Type Conversion17/1
  Data Type Conversion17/1 -> Mux/10
  [Test10] -> Data Type Conversion19/1
  [Test9] -> Data Type Conversion18/1
  Data Type Conversion18/1 -> Mux1/9
  Data Type Conversion19/1 -> Mux1/10
  StringDelete10/1 -> [Baseline11], StringDisplay10/1
  StringDelete10/2 -> [Baseline12], Display10/1
  StringDelete11/1 -> [Test11], StringDisplay11/1
  StringDelete11/2 -> Display11/1, [Test12]
  Constant10/1 -> StringDelete11/2, StringDelete10/2
  Constant11/1 -> StringDelete11/3, StringDelete10/3
  StringSource2/1 -> StringDelete11/1, StringDelete10/1
  [Baseline11] -> Data Type Conversion20/1
  Data Type Conversion20/1 -> Mux/11
  [Baseline12] -> Data Type Conversion21/1
  Data Type Conversion21/1 -> Mux/12
  [Test12] -> Data Type Conversion23/1
  [Test11] -> Data Type Conversion22/1
  Data Type Conversion22/1 -> Mux1/11
  Data Type Conversion23/1 -> Mux1/12
  StringDelete12/1 -> [Baseline13], StringDisplay12/1
  StringDelete12/2 -> [Baseline14], Display12/1
  StringDelete13/1 -> [Test13], StringDisplay13/1
  StringDelete13/2 -> Display13/1, [Test14]
  Constant12/1 -> StringDelete13/2, StringDelete12/2
  Constant13/1 -> StringDelete13/3, StringDelete12/3
  StringSource3/1 -> StringDelete13/1, StringDelete12/1
  [Baseline13] -> Data Type Conversion24/1
  Data Type Conversion24/1 -> Mux/13
  [Baseline14] -> Data Type Conversion25/1
  Data Type Conversion25/1 -> Mux/14
  [Test14] -> Data Type Conversion27/1
  [Test13] -> Data Type Conversion26/1
  Data Type Conversion26/1 -> Mux1/13
  Data Type Conversion27/1 -> Mux1/14
  StringDelete14/1 -> [Baseline15], StringDisplay14/1
  StringDelete14/2 -> [Baseline16], Display14/1
  StringDelete15/1 -> [Test15], StringDisplay15/1
  StringDelete15/2 -> Display15/1, [Test16]
  Constant14/1 -> StringDelete15/2, StringDelete14/2
  Constant15/1 -> StringDelete15/3, StringDelete14/3
  StringSource4/1 -> StringDelete15/1, StringDelete14/1
  [Test16] -> Data Type Conversion29/1
  [Test15] -> Data Type Conversion28/1
  Data Type Conversion28/1 -> Mux1/15
  Data Type Conversion29/1 -> Mux1/16
  [Baseline15] -> Data Type Conversion30/1
  Data Type Conversion30/1 -> Mux/15
  [Baseline16] -> Data Type Conversion31/1
  Data Type Conversion31/1 -> Mux/16

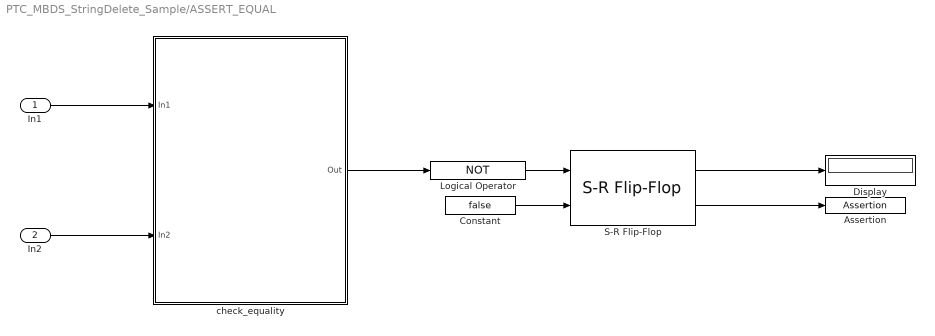
== system PTC_MBDS_StringDelete_Sample/ASSERT_EQUAL ==
  In1 : Inport
  In2 : Inport  Port=2
  Assertion : Assertion
  Constant : Constant  Value=false
  Display : Display
  Logical Operator : Logic  Operator=NOT  AllPortsSameDT=off  OutDataTypeStr=boolean
  S-R Flip-Flop : simulink_extras/Flip Flops/S-R Flip-Flop  initial_condition=0
  check_equality : MATLAB Function  TreatAsAtomicUnit=on
  wires:
  S-R Flip-Flop/1 -> Display/1
  check_equality/1(Out) -> Logical Operator/1
  Constant/1 -> S-R Flip-Flop/2
  S-R Flip-Flop/2 -> Assertion/1
  In2/1 -> check_equality/2(In2)
  In1/1 -> check_equality/1(In1)
  Logical Operator/1 -> S-R Flip-Flop/1

== matlab function PTC_MBDS_StringDelete_Sample/ASSERT_EQUAL/check_equality ==
  data: In1 input; Out output; In2 input
function Out = check_equality(In1, In2)
%#codegen

Out = isequaln(In1, In2);

end
